simulink model "vehiclemodel_simple_empty_2020a"  (R2023b)
settings: Solver=ode23tb  StartTime=0.0  StopTime=20  FixedStep=.001  MaxStep=0.001  RelTol=1e-3  EnableMultiTasking=on
values from neighbouring files (symbols this model uses):
  a = 1.5    [truck_data_test.m]
  Ab = 0.01    [truck_data_test.m]
  ARV = 4    [truck_data_test.m]
  b = 3    [truck_data_test.m]
  Bh = 5    [truck_data_test.m]
  Bs = 10    [truck_data_test.m]
  CDV = 0.7    [truck_data_test.m]
  Ch = 2*1.2    (= 2.4)    [truck_data_test.m]
  Cs = 1.9*1.2    (= 2.28)    [truck_data_test.m]
  Dh = 0.3    [truck_data_test.m]
  Ds = 1    [truck_data_test.m]
  Eh = 1    [truck_data_test.m]
  Es = 0.97    [truck_data_test.m]
  fa = 1    [truck_data_test.m]
  ff = 1    [truck_data_test.m]
  g = 9.81    [truck_data_test.m]
  hs = 0.20    (= 0.2)    [truck_data_test.m]
  Ms = 7000    [truck_data_test.m]
  nm = 1    [truck_data_test.m]
  ntire = 10    [truck_data_test.m]
  P_s = 8e5    (= 800000)    [truck_data_test.m]
  Patm = 101356    [truck_data_test.m]
  Po = 50e3    (= 50000)    [truck_data_test.m]
  pr = 1.225    [truck_data_test.m]
  rs1 = rw1    (= 0.4)    [truck_data_test.m]
  Rw = rw1    (= 0.4)    [truck_data_test.m]
  T = 2.5    [truck_data_test.m]
  Vox = intVEL    (= 20)    [truck_data_test.m]
  WBF = 4    [truck_data_test.m]
  wp = 1/(2*(tan(wang/2)))    [truck_data_test.m]
  wr = 0.4    [truck_data_test.m]
  Xtire = 20    [truck_data_test.m]
settings Model: Creator=Abdul Moiz Awan  LastModifiedBy=yusufcagriogut
settings SolverCC: ZeroCrossControl=EnableAll  ZeroCrossAlgorithm=Adaptive  AlgebraicLoopSolver=TrustRegion
settings DataIOCC: LimitDataPoints=on  MaxDataPoints=10000
settings OptimizationCC: LifeSpan=inf
settings DebuggingCC: UnconnectedInputMsg=warning  UnconnectedOutputMsg=warning  UnconnectedLineMsg=warning  AllowSymbolicDim=off  SFUnexpectedBacktrackingDiag=warning  SFNoUnconditionalDefaultTransitionDiag=warning  SFExecutionAtInitializationDiag=none  ArithmeticOperatorsInVariantConditions=warning
settings ModelReferenceCC: EnableRefExpFcnMdlSchedulingChecks=on
settings SFSimCC: SimUseLocalCustomCode=off  CustomCodeUndefinedFunction=UseInterfaceOnly
settings RTWCC: RTWUseLocalCustomCode=off
settings CodeAppCC: StateflowObjectComments=on
settings GRTTargetCC: TargetLangStandard=C89/C90 (ANSI)
settings ConfigComp: CovMetricSettings=dw  CovSaveCumulativeToWorkspaceVar=on  CovSaveSingleToWorkspaceVar=on  CovExternalEMLEnable=off  CovSFcnEnable=off
settings SimscapeCC: SimscapeLogType=all  SimscapeLogSimulationStatistics=on  SimscapeLogDataHistory=10000

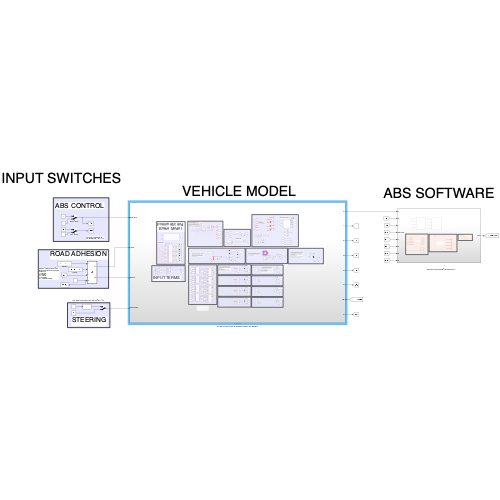
[thumbnail: Simulink's stored preview of the top-level diagram]
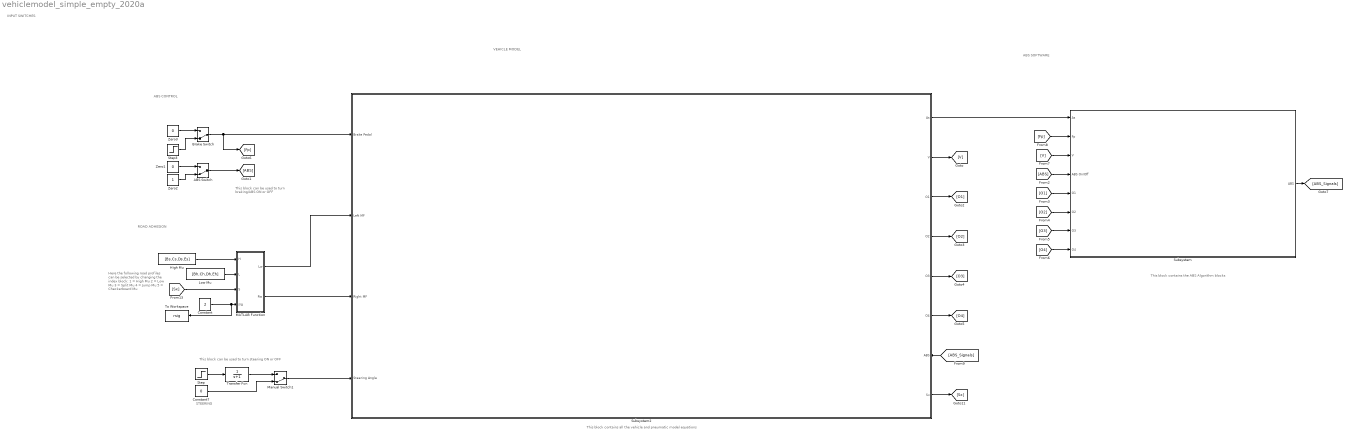
== system vehiclemodel_simple_empty_2020a ==
  note: Here the following road profiles
      | can be selected by changing the
      | index block:
      | 1 = High Mu
      | 2 = Low Mu
      | 3 = Split Mu
      | 4 = Jump Mu
      | 5 = Checkerboard Mu
  note: ABS CONTROL
  note: VEHICLE MODEL
  note: ROAD ADHESION
  note: ABS SOFTWARE
  note: INPUT SWITCHES
  note: STEERING
  note: This block contains the ABS Algorithm blocks
  note: This block contains all the vehicle and pneumatic model equations
  note: This block can be used to turn steering ON or OFF
  note: This block can be used to
      | turn braking/ABS ON or OFF
  ABS Switch : ManualSwitch  CurrentSetting=0
  Brake Switch : ManualSwitch  CurrentSetting=0
  Constant : Constant  Value=2
  Constant7 : Constant  Value=0
  High Mu : Constant  Value=[Bs,Cs,Ds,Es]
  Low Mu : Constant  Value=[Bh,Ch,Dh,Eh]
  MATLAB Function : MATLAB Function  TreatAsAtomicUnit=on
  Manual Switch1 : ManualSwitch  CurrentSetting=0
  Step : Step  After=deg2rad(3)  SampleTime=0
  Step3 : Step  SampleTime=0
  Subsystem : Subsystem
  Subsystem2 : Subsystem
      settings: PortSchema="{\"entries\":[{\"content\":{\"sides\":[{\"content\":{\"connectorIds\":[\"In1\",\"In2\",\"In3\",\"In4\"]},\"type\":\"ConnectorPlacement.EquallySpacedRectSide\",\"uuid\":\"8e59d40e-014f-4f71-bd3c-8a56eaa9320b\"},{\"content\":{\"connectorIds\":[\"Out1\",\"Out2\",\"Out3\",\"Out4\",\"Out5\",\"Out6\",\"In5\",\"Out7\"],\"side\":\"RIGHT\"},\"type\":\"ConnectorPlacement.EquallySpacedRectSide\",\"uuid\":\"f787145f-ddea-4867-9ee8-cb71aff46f3c\"},{\"content\":{\"side\":\"TOP\"},\"type\":\"ConnectorPlacement.EquallySpacedRectSide\",\"uuid\":\"5155c75c-b431-498b-ab23-6aa92088c174\"},{\"content\":{\"side\":\"BOTTOM\"},\"type\":\"ConnectorPlacement.EquallySpacedRectSide\",\"uuid\":\"2f8d0388-20b7-4bc4-84a6-56d75173057c\"}]},\"type\":\"ConnectorPlacement.EquallySpacedConnector\",\"uuid\":\"a4266be2-998a-4783-9e32-f9f9cb8c25f7\"}],\"packageUris\":[\"http://schema.mathworks.com/mf0/Connector/R2020b\"],\"version\":\"1.0\"}"
  To Workspace : ToWorkspace  VariableName=rsig  SaveFormat=Timeseries  SampleTime=-1
  Transfer Fcn : TransferFcn  Denominator=[1 1]
  Zero1 : Constant  Value=0  OutDataTypeStr=Inherit: Inherit via back propagation
  Zero2 : Constant  OutDataTypeStr=Inherit: Inherit via back propagation
  Zero3 : Constant  Value=0  OutDataTypeStr=Inherit: Inherit via back propagation
  wires:
  Zero3/1 -> Brake Switch/1
  Brake Switch/1 -> [Fp], Subsystem2/1(Brake Pedal)
  Zero1/1 -> ABS Switch/1
  Zero2/1 -> ABS Switch/2
  Step3/1 -> Brake Switch/2
  Subsystem2/2(V) -> [V]
  ABS Switch/1 -> [ABS]
  [ABS] -> Subsystem/4(ABS On/Off)
  Subsystem2/3(O1) -> [O1]
  Subsystem2/4(O2) -> [O2]
  Subsystem2/5(O3) -> [O3]
  Subsystem2/6(O4) -> [O4]
  [O1] -> Subsystem/5(O1)
  [O2] -> Subsystem/6(O2)
  [O3] -> Subsystem/7(O3)
  [O4] -> Subsystem/8(O4)
  [V] -> Subsystem/3(V)
  [Fp] -> Subsystem/2(Fp)
  Subsystem/1(ABS) -> [ABS_Signals]
  [ABS_Signals] -> Subsystem2/5(ABS)
  Step/1 -> Transfer Fcn/1
  Constant7/1 -> Manual Switch1/2
  Transfer Fcn/1 -> Manual Switch1/1
  Manual Switch1/1 -> Subsystem2/4(Steering Angle)
  MATLAB Function/2(Rw) -> Subsystem2/3(Right MF)
  Subsystem2/7(Sx) -> [Sx]
  Subsystem2/1(As) -> Subsystem/1(As)
  High Mu/1 -> MATLAB Function/1(H)
  Low Mu/1 -> MATLAB Function/2(L)
  [Sx] -> MATLAB Function/3(S)
  Constant/1 -> To Workspace/1, MATLAB Function/4(sig)
  MATLAB Function/1(Lw) -> Subsystem2/2(Left MF)

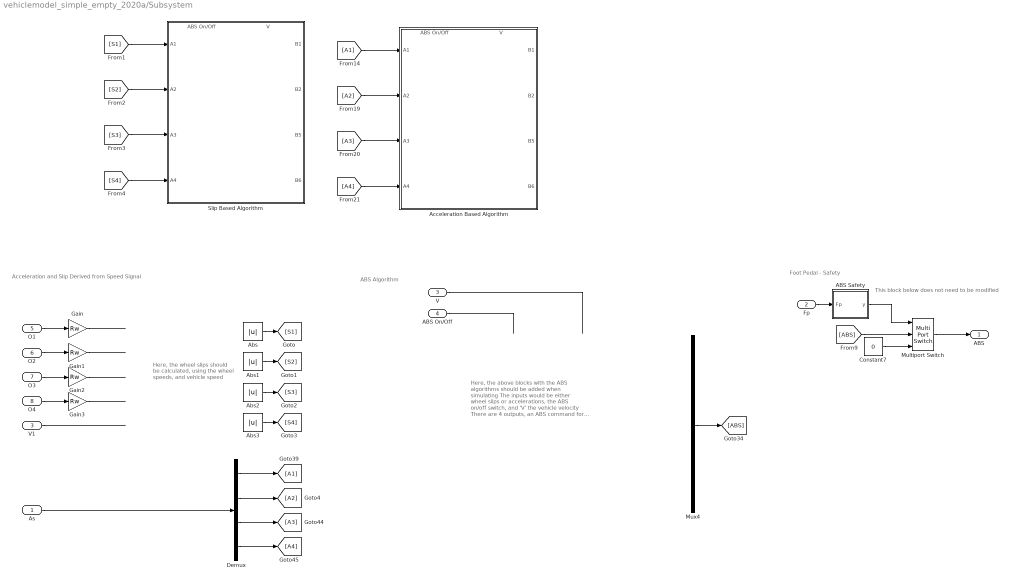
== system vehiclemodel_simple_empty_2020a/Subsystem ==
  note: Here, the wheel slips
      | should be calculated,
      | using the wheel speeds,
      | and vehicle speed
  note: Foot Pedal - Safety
  note: Acceleration and Slip Derived from Speed Signal
  note: ABS Algorithm
  note: Here, the above blocks
      | with the ABS algorithms
      | should be added when simulating
      |
      | The inputs would be either wheel
      | slips or accelerations, the ABS on/off
      | switch, and 'V' the vehicle velocity
      |
      | There are 4 outputs, an ABS command
      | for each wheel
  note: This block below does not need to be modified
  As : Inport
  Fp : Inport  Port=2
  V : Inport  Port=3
  ABS On/Off : Inport  Port=4
  O1 : Inport  Port=5
  O2 : Inport  Port=6
  O3 : Inport  Port=7
  O4 : Inport  Port=8
  ABS Safety : MATLAB Function  TreatAsAtomicUnit=on
  Abs{,1..3} (4 alike) : Abs  SaturateOnIntegerOverflow=off
  Acceleration Based Algorithm : Subsystem
      settings: PortSchema="{\"entries\":[{\"content\":{\"sides\":[{\"content\":{\"connectorIds\":[\"In1\",\"In2\",\"In3\",\"In4\"]},\"type\":\"ConnectorPlacement.EquallySpacedRectSide\",\"uuid\":\"0cf54bfd-7e95-4e49-acd0-cde280c9a58c\"},{\"content\":{\"connectorIds\":[\"Out1\",\"Out2\",\"Out3\",\"Out4\"],\"side\":\"RIGHT\"},\"type\":\"ConnectorPlacement.EquallySpacedRectSide\",\"uuid\":\"586cf5cf-8639-456b-b48e-ff3e77509e66\"},{\"content\":{\"connectorIds\":[\"In5\",\"In6\"],\"side\":\"TOP\"},\"type\":\"ConnectorPlacement.EquallySpacedRectSide\",\"uuid\":\"7bf15eda-a81d-4bd7-ab4e-9ac22b0c7db2\"}]},\"type\":\"ConnectorPlacement.EquallySpacedConnector\",\"uuid\":\"c618e342-5041-438f-9a1b-df95de83ed7e\"}],\"packageUris\":[\"http://schema.mathworks.com/mf0/Connector/R2020b\"],\"version\":\"1.0\"}"
  Constant7 : Constant  Value=0
  Demux : Demux
  Gain{,1..3} (4 alike) : Gain  Gain=Rw
  Multiport Switch : MultiPortSwitch  Inputs=2  SaturateOnIntegerOverflow=off  InputSameDT=off
  Mux4 : Mux
  Slip Based Algorithm : Subsystem
      settings: PortSchema="{\"entries\":[{\"content\":{\"sides\":[{\"content\":{\"connectorIds\":[\"In1\",\"In2\",\"In3\",\"In4\"]},\"type\":\"ConnectorPlacement.EquallySpacedRectSide\",\"uuid\":\"0cf54bfd-7e95-4e49-acd0-cde280c9a58c\"},{\"content\":{\"connectorIds\":[\"Out1\",\"Out2\",\"Out3\",\"Out4\"],\"side\":\"RIGHT\"},\"type\":\"ConnectorPlacement.EquallySpacedRectSide\",\"uuid\":\"586cf5cf-8639-456b-b48e-ff3e77509e66\"},{\"content\":{\"connectorIds\":[\"In5\",\"In6\"],\"side\":\"TOP\"},\"type\":\"ConnectorPlacement.EquallySpacedRectSide\",\"uuid\":\"7bf15eda-a81d-4bd7-ab4e-9ac22b0c7db2\"}]},\"type\":\"ConnectorPlacement.EquallySpacedConnector\",\"uuid\":\"c618e342-5041-438f-9a1b-df95de83ed7e\"}],\"packageUris\":[\"http://schema.mathworks.com/mf0/Connector/R2020b\"],\"version\":\"1.0\"}"
  V1 : InportShadow  Port=3
  ABS : Outport
  wires:
  V/1 -> ?
  ? -> Mux4/4
  ? -> Mux4/2
  ABS On/Off/1 -> ?
  [ABS] -> Multiport Switch/2
  ? -> Mux4/1
  Mux4/1 -> [ABS]
  ? -> Mux4/3
  Constant7/1 -> Multiport Switch/3
  ABS Safety/1(y) -> Multiport Switch/1
  Fp/1 -> ABS Safety/1(Fp)
  Multiport Switch/1 -> ABS/1
  V1/1 -> ?
  Gain/1 -> ?
  Gain1/1 -> ?
  Gain2/1 -> ?
  Gain3/1 -> ?
  Abs/1 -> [S1]
  Abs1/1 -> [S2]
  Abs2/1 -> [S3]
  Demux/4 -> [A4]
  O4/1 -> Gain3/1
  Demux/1 -> [A1]
  O1/1 -> Gain/1
  O2/1 -> Gain1/1
  O3/1 -> Gain2/1
  Demux/2 -> [A2]
  Demux/3 -> [A3]
  As/1 -> Demux/1
  [A4] -> Acceleration Based Algorithm/4(A4)
  [A3] -> Acceleration Based Algorithm/3(A3)
  [A2] -> Acceleration Based Algorithm/2(A2)
  [A1] -> Acceleration Based Algorithm/1(A1)
  Abs3/1 -> [S4]
  [S1] -> Slip Based Algorithm/1(A1)
  [S2] -> Slip Based Algorithm/2(A2)
  [S3] -> Slip Based Algorithm/3(A3)
  [S4] -> Slip Based Algorithm/4(A4)

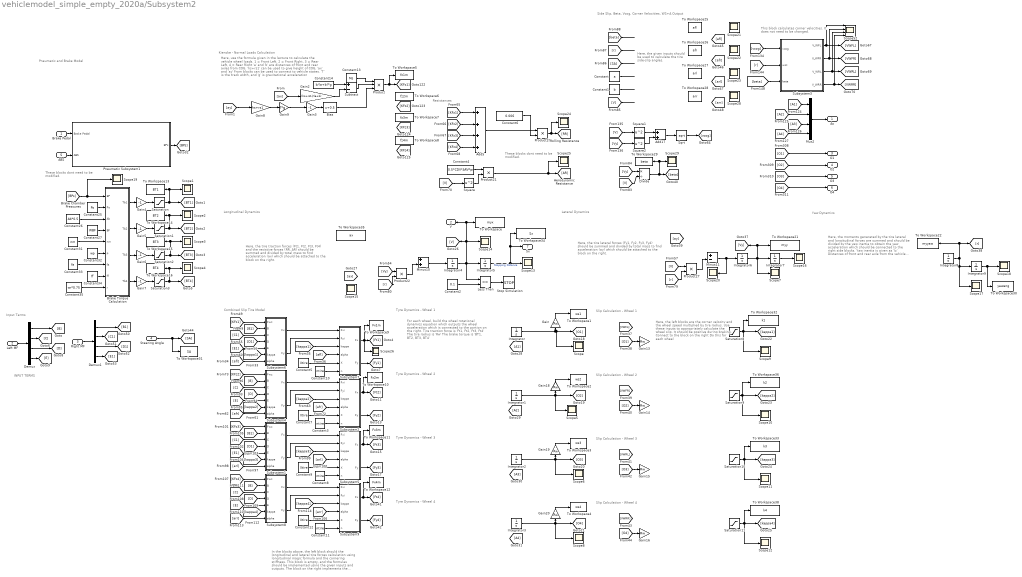
== system vehiclemodel_simple_empty_2020a/Subsystem2 ==
  note: This block calculates corner velocities.
      | It does not need to be changed.
  note: These blocks dont
      | need to be modified.
  note: Combined Slip Tire Model
  note: Side Slip, Beta, Vcog, Corner Velocities, WS+A Output
  note: Yaw Dynamics
  note: Lateral Dynamics
  note: Resistances
  note: Input Terms
  note: Pneumatic and Brake Model
  note: INPUT TERMS
  note: Kiencke - Normal Loads Calculation
  note: Tyre Dynamics - Wheel 1
  note: Tyre Dynamics - Wheel 2
  note: Tyre Dynamics - Wheel 3
  note: Tyre Dynamics - Wheel 4
  note: Slip Calculation - Wheel 1
  note: Slip Calculation - Wheel 2
  note: Slip Calculation - Wheel 3
  note: Slip Calculation - Wheel 4
  note: Longitudinal Dynamics
  note: In the blocks above, the left block should
      | the longitudinal and lateral tire forces calculation
      | using longitudinal magic formula and the
      | cornering stiffness. This block is empty, and the
      | formulas should be implemented using the given
      | inputs and outputs.
      |
      | The block on the right implements the combined
      | slip model and does not need to be modified.
  note: For each wheel, build the wheel rotational
      | dynamics equation which outputs the wheel
      | acceleration which is connected to the portion
      | on the right.
      |
      | Tire traction force is 'Ft1, Ft2, Ft3, Ft4'
      | The tire radius is 'Rw'
      | The brake torque is 'BT1, BT2, BT3, BT4'
  note: Here, the left blocks are the corner velocity
      | and the wheel speed multiplied by tire
      | radius. Use these inputs to appropriately
      | calculate the wheel slip.
      |
      | It should be positive during braking. Connect
      | to the block on the right
      |
      | Do this for each wheel
  note: Here, the tire traction forces (Ft1, Ft2, Ft3, Ft4)
      | and the resistive forces (RR, AR) should be
      | summed and divided by total mass to find
      | acceleration (ax) which should be attached to
      | the block on the right.
  note: Here, the tire lateral forces (Fy1, Fy2, Fy3, Fy4)
      | should be summed and divided by total mass
      | to find acceleration (ay) which should be attached
      | to the block on the right.
  note: Here, the moments generated by the tire lateral
      | and longitudinal forces are summed and should
      | be divided by the yaw inertia to obtain the yaw
      | acceleration which should be connected to the
      | right side blocks.
      |
      | Yaw inertia is given as 'Iz'
      |
      | Distances of front and rear axle from the vehicle
      | COG are given as 'a' and 'b' respectively.
  note: Here, use the formula given in the lecture to
      | calculate the vehicle wheel loads.
      | 1 = Front Left, 2 = Front Right, 3 = Rear Left, 4 = Rear Right
      |
      | 'a' and 'b' are distances of front and rear axles from COG,
      | 'hs+rs1' can be used to give height of COG,
      | 'ax' and 'ay' From blocks can be used to connect to vehicle
      | states.
      | 'T' is the track width, and 'g' is gravitational acceleration
  note: These blocks dont
      | need to be modified.
  note: Here, the given
      | inputs should
      | be used to calculate
      | the tire side-slip angles.
  Brake Pedal : Inport
  Left MF : Inport  Port=2
  Right MF : Inport  Port=3
  Steering Angle : Inport  Port=4
  ABS : Inport  Port=5
  Add17 : Sum
  Add5 : Sum  Inputs=++++
  Bias : Bias  Bias=0.5  SaturateOnIntegerOverflow=off
  Brake Torque Calculation : MATLAB Function  TreatAsAtomicUnit=on
  Constant : Constant  Value=a
  Constant1 : Constant  Value=b
  Constant{3,8,10..11} (4 alike) : Constant  Value=ntire
  Constant{5,7,9,12} (4 alike) : Constant  Value=Xtire
  Constant13 : Constant  Value=Ms
  Constant14 : Constant  Value=b/(a+b)*g
  Constant2 : Constant  Value=0.1
  Constant25 : Constant  Value=Po
  Constant26 : Constant  Value=Ab*0.5
  Constant27 : Constant  Value=WBF
  Constant31 : Constant  Value=nm
  Constant32 : Constant  Value=wp
  Constant33 : Constant  Value=fa
  Constant34 : Constant  Value=ff
  Constant35 : Constant  Value=wr*0.75
  Constant4 : Constant  Value=0.5*CDV*ARV*pr
  Constant6 : Constant  Value=0.006
  Demux : Demux
  Demux1 : Demux
  Divide : Product  Inputs=*/
  Gain{,13..16,18..20} (8 alike) : Gain  Gain=Rw
  Gain2 : Gain  Gain=(hs+rs1)/(a+b)
  Gain{3..7} (5 alike) : Gain  Gain=-1
  Gain8 : Gain  Gain=hs+rs1
  Gain9 : Gain  Gain=T*g
  Integrator{,1..3} (4 alike) : Integrator  InitialCondition=Vox/Rw  LimitOutput=on  LowerSaturationLimit=0
  Integrator4 : Integrator  InitialCondition=Vox
  Integrator{5..9} (5 alike) : Integrator
  Less Than : RelationalOperator  Operator=<=  OutDataTypeStr=boolean  RndMeth=Simplest  InputSameDT=off
  Minus10 : Sum
  Minus11 : Sum  Inputs=+-
  Mux2 : Mux
  Pneumatic Subsystem1 : Subsystem
  Product : Product  Inputs=3
  Product{20..22,27} (4 alike) : Product
  Saturation{,1..3} (4 alike) : Saturate  UpperLimit=0  LowerLimit=-inf
  Saturation{8..11} (4 alike) : Saturate  UpperLimit=1  LowerLimit=-1
  Scope{,1..26,28..29} (29 alike) : Scope
  Scope52 : Scope  NumInputPorts=4
  Sqrt : Sqrt
  Square : Math  Operator=square
  Square1 : Math  Operator=square
  Square2 : Math  Operator=square
  Stop Simulation : Stop
  Subsystem1 : Subsystem
  Subsystem2 : Subsystem
  Subsystem3 : Subsystem
  Subsystem4 : Subsystem
  Subsystem5 : Subsystem
  Subsystem6 : Subsystem
  Subsystem7 : Subsystem
  Subsystem8 : Subsystem
  Subsystem9 : Subsystem
  Subtract : Sum  Inputs=+-
  To Workspace : ToWorkspace  VariableName=myx  SaveFormat=Timeseries  SampleTime=-1
  To Workspace1 : ToWorkspace  VariableName=ws1  SaveFormat=Timeseries  SampleTime=-1
  To Workspace10 : ToWorkspace  VariableName=Fx2m  SaveFormat=Timeseries  SampleTime=-1
  To Workspace11 : ToWorkspace  VariableName=Fx3m  SaveFormat=Timeseries  SampleTime=-1
  To Workspace12 : ToWorkspace  VariableName=Fx4m  SaveFormat=Timeseries  SampleTime=-1
  To Workspace13 : ToWorkspace  VariableName=BT1  SaveFormat=Timeseries  SampleTime=-1
  To Workspace14 : ToWorkspace  VariableName=BT2  SaveFormat=Timeseries  SampleTime=-1
  To Workspace15 : ToWorkspace  VariableName=BT3  SaveFormat=Timeseries  SampleTime=-1
  To Workspace16 : ToWorkspace  VariableName=BT4  SaveFormat=Timeseries  SampleTime=-1
  To Workspace2 : ToWorkspace  VariableName=ws2  SaveFormat=Timeseries  SampleTime=-1
  To Workspace21 : ToWorkspace  VariableName=myy  SaveFormat=Timeseries  SampleTime=-1
  To Workspace22 : ToWorkspace  VariableName=myyaw  SaveFormat=Timeseries  SampleTime=-1
  To Workspace25 : ToWorkspace  VariableName=afl  SaveFormat=Timeseries  SampleTime=-1
  To Workspace26 : ToWorkspace  VariableName=afr  SaveFormat=Timeseries  SampleTime=-1
  To Workspace27 : ToWorkspace  VariableName=arl  SaveFormat=Timeseries  SampleTime=-1
  To Workspace28 : ToWorkspace  VariableName=arr  SaveFormat=Timeseries  SampleTime=-1
  To Workspace29 : ToWorkspace  VariableName=beta  SaveFormat=Timeseries  SampleTime=-1
  To Workspace3 : ToWorkspace  VariableName=ws3  SaveFormat=Timeseries  SampleTime=-1
  To Workspace30 : ToWorkspace  VariableName=yawang  SaveFormat=Timeseries  SampleTime=-1
  To Workspace31 : ToWorkspace  VariableName=SA  SaveFormat=Timeseries  SampleTime=-1
  To Workspace32 : ToWorkspace  VariableName=k1  SaveFormat=Timeseries  SampleTime=-1
  To Workspace33 : ToWorkspace  VariableName=k3  SaveFormat=Timeseries  SampleTime=-1
  To Workspace34 : ToWorkspace  VariableName=Sx  SaveFormat=Timeseries  SampleTime=-1
  To Workspace35 : ToWorkspace  VariableName=ax  SaveFormat=Timeseries  SampleTime=-1
  To Workspace36 : ToWorkspace  VariableName=k2  SaveFormat=Timeseries  SampleTime=-1
  To Workspace38 : ToWorkspace  VariableName=k4  SaveFormat=Timeseries  SampleTime=-1
  To Workspace4 : ToWorkspace  VariableName=ws4  SaveFormat=Timeseries  SampleTime=-1
  To Workspace5 : ToWorkspace  VariableName=fz1m  SaveFormat=Timeseries  SampleTime=-1
  To Workspace6 : ToWorkspace  VariableName=fz2m  SaveFormat=Timeseries  SampleTime=-1
  To Workspace7 : ToWorkspace  VariableName=fz3m  SaveFormat=Timeseries  SampleTime=-1
  To Workspace8 : ToWorkspace  VariableName=fz4m  SaveFormat=Timeseries  SampleTime=-1
  To Workspace9 : ToWorkspace  VariableName=Fx1m  SaveFormat=Timeseries  SampleTime=-1
  As : Outport
  V : Outport  Port=2
  O1 : Outport  Port=3
  O2 : Outport  Port=4
  O3 : Outport  Port=5
  O4 : Outport  Port=6
  Sx : Outport  Port=7
  wires:
  Brake Pedal/1 -> Pneumatic Subsystem1/1(Brake Pedal)
  ? -> To Workspace8/1, [KFz4]
  ? -> To Workspace7/1, [KFz3]
  ? -> To Workspace6/1, [KFz2]
  Brake Torque Calculation/4(Tb4) -> Gain7/1
  Gain5/1 -> Saturation1/1
  Gain4/1 -> Saturation/1
  Constant27/1 -> Brake Torque Calculation/4(BF)
  Constant26/1 -> Brake Torque Calculation/3(Ab)
  Gain6/1 -> Saturation2/1
  Brake Torque Calculation/3(Tb3) -> Gain6/1
  Constant31/1 -> Brake Torque Calculation/5(nm)
  Constant33/1 -> Brake Torque Calculation/7(fa)
  Gain7/1 -> Saturation3/1
  Constant35/1 -> Brake Torque Calculation/9(r)
  Brake Torque Calculation/1(Tb1) -> Gain4/1
  Constant32/1 -> Brake Torque Calculation/6(p)
  Brake Torque Calculation/2(Tb2) -> Gain5/1
  Constant25/1 -> Brake Torque Calculation/2(Po)
  Constant34/1 -> Brake Torque Calculation/8(ff)
  Saturation/1 -> [BT1], Scope1/1, To Workspace13/1
  Saturation1/1 -> [BT2], Scope2/1, To Workspace14/1
  Saturation3/1 -> [BT4], Scope4/1, To Workspace16/1
  Pneumatic Subsystem1/1(BPs) -> [BPs]
  Left MF/1 -> Demux/1
  Demux/1 -> [B]
  Demux/2 -> [C]
  Demux/3 -> [D]
  Demux/4 -> [E]
  Integrator/1 -> [O1], Scope/1, Gain/1
  ? -> [A1], Integrator/1
  ? -> Integrator1/1, [A2]
  Integrator1/1 -> [O2], Scope5/1, Gain18/1
  Integrator2/1 -> [O3], Scope6/1, Gain19/1
  ? -> Integrator2/1, [A3]
  ? -> Integrator3/1, [A4]
  Integrator3/1 -> [O4], Scope8/1, Gain20/1
  Saturation8/1 -> Scope9/1, To Workspace32/1, [kappa1]
  [O1] -> Gain13/1
  [O2] -> Gain14/1
  Saturation9/1 -> To Workspace36/1, Scope10/1, [kappa2]
  Saturation10/1 -> Scope11/1, To Workspace33/1, [kappa3]
  [O3] -> Gain15/1
  [O4] -> Gain16/1
  Saturation11/1 -> To Workspace38/1, Scope12/1, [kappa4]
  Integrator5/1 -> To Workspace34/1, Sx/1, Scope13/1  "Stopping Dstance"
  Less Than/1 -> Stop Simulation/1
  Constant2/1 -> Less Than/2
  Integrator4/1 -> Less Than/1, To Workspace/1, V/1, Scope14/1, [V], Integrator5/1
  ? -> To Workspace35/1, Scope15/1, [ax], Minus10/1
  Gain/1 -> To Workspace1/1
  Gain18/1 -> To Workspace2/1
  Gain19/1 -> To Workspace3/1
  Gain20/1 -> To Workspace4/1
  Add5/1 -> Product20/1
  [KFz4] -> Add5/4
  [KFz3] -> Add5/3
  [KFz2] -> Add5/2
  [KFz1] -> Add5/1
  Product20/1 -> Scope24/1, [RR]
  Constant4/1 -> Product21/1
  [V] -> Square/1
  Square/1 -> Product21/2
  Product21/1 -> Scope25/1, [AR]
  Constant6/1 -> Product20/2
  Product/1 -> To Workspace5/1, [KFz1]
  [O3] -> O3/1
  [O2] -> O2/1
  [O4] -> O4/1
  [O1] -> O1/1
  ABS/1 -> Pneumatic Subsystem1/2(ABS)
  Product22/1 -> Minus10/2
  Product27/1 -> Minus11/2
  ? -> Minus11/1, [ay]
  Minus11/1 -> Scope20/1, Integrator6/1
  Integrator6/1 -> To Workspace21/1, [Vy], Scope7/1, Integrator7/1
  Integrator7/1 -> Scope16/1
  [Vy] -> Product22/1
  [V] -> Product27/1
  ? -> Integrator8/1
  Integrator8/1 -> Scope17/1, Integrator9/1, To Workspace22/1, [r]
  Integrator9/1 -> Scope18/1, To Workspace30/1
  [r] -> Product27/2
  [r] -> Product22/2
  [Vy] -> Divide/1
  [V] -> Divide/2
  Divide/1 -> Scope29/1, To Workspace29/1, [beta]
  Steering Angle/1 -> To Workspace31/1, [SA]
  Constant/1 -> ?
  Constant1/1 -> ?
  [V] -> ?
  [SA] -> ?
  [r] -> ?
  [beta] -> ?
  ? -> To Workspace25/1, Scope21/1, [afl]  "From Formula"
  ? -> To Workspace26/1, Scope22/1, [afr]  "From Fomula"
  ? -> To Workspace27/1, Scope23/1, [arl]  "From Formula"
  ? -> Scope28/1, To Workspace28/1, [arr]  "From Formula"
  Right MF/1 -> Demux1/1
  Minus10/1 -> Integrator4/1
  [BPs] -> Scope19/1, Brake Torque Calculation/1(BP)
  [A2] -> Mux2/2
  [A1] -> Mux2/1
  [A3] -> Mux2/3
  [A4] -> Mux2/4
  Mux2/1 -> As/1
  Subsystem3/4(V_WRR) -> Scope52/4, [VWRR]
  Subsystem3/2(V_WFR) -> Scope52/2, [VWFR]
  [vcog] -> Subsystem3/1(vcog)
  [r] -> Subsystem3/2(wsz)
  [beta] -> Subsystem3/3(beta)
  Subsystem3/3(V_WRL) -> Scope52/3, [VWRL]
  Subsystem3/1(V_WFL) -> Scope52/1, [VWFL]
  [V] -> Square1/1
  [Vy] -> Square2/1
  Square1/1 -> Add17/1
  Square2/1 -> Add17/2
  Add17/1 -> Sqrt/1
  Sqrt/1 -> [vcog]
  Demux1/1 -> [B1]
  Demux1/2 -> [C1]
  Demux1/3 -> [D1]
  Demux1/4 -> [E1]
  [afl] -> Subsystem7/4(alpha)
  Subsystem6/2(Fy) -> Subsystem7/2(Fyi)
  [kappa1] -> Subsystem7/3(kappa)
  Subsystem7/2(Fy) -> [Fy1]
  [C1] -> Subsystem6/3(C)
  [kappa1] -> Subsystem6/6(kappa)
  [D1] -> Subsystem6/4(D)
  [KFz1] -> Subsystem6/1(Fwz)
  [E1] -> Subsystem6/5(E)
  Constant5/1 -> Subsystem7/5(X)
  [afl] -> Subsystem6/7(alpha)
  Subsystem6/1(Fx) -> Subsystem7/1(Fxi)
  [B1] -> Subsystem6/2(B)
  Constant10/1 -> Subsystem7/6(n)
  Constant3/1 -> Subsystem2/6(n)
  [B] -> Subsystem4/2(B)
  Subsystem2/1(Fx) -> To Workspace10/1, [Ft2]
  Subsystem4/1(Fx) -> Subsystem2/1(Fxi)
  [afr] -> Subsystem4/7(alpha)
  Constant7/1 -> Subsystem2/5(X)
  [E] -> Subsystem4/5(E)
  [KFz2] -> Subsystem4/1(Fwz)
  [D] -> Subsystem4/4(D)
  [kappa2] -> Subsystem4/6(kappa)
  [C] -> Subsystem4/3(C)
  Subsystem2/2(Fy) -> [Fy2]
  [kappa2] -> Subsystem2/3(kappa)
  Subsystem4/2(Fy) -> Subsystem2/2(Fyi)
  [afr] -> Subsystem2/4(alpha)
  [arl] -> Subsystem5/4(alpha)
  Subsystem1/2(Fy) -> Subsystem5/2(Fyi)
  [kappa3] -> Subsystem5/3(kappa)
  Subsystem5/2(Fy) -> [Fy3]
  [C1] -> Subsystem1/3(C)
  [kappa3] -> Subsystem1/6(kappa)
  [D1] -> Subsystem1/4(D)
  [KFz3] -> Subsystem1/1(Fwz)
  [E1] -> Subsystem1/5(E)
  Constant9/1 -> Subsystem5/5(X)
  [arl] -> Subsystem1/7(alpha)
  Subsystem1/1(Fx) -> Subsystem5/1(Fxi)
  Subsystem5/1(Fx) -> To Workspace11/1, [Ft3]
  [B1] -> Subsystem1/2(B)
  Constant8/1 -> Subsystem5/6(n)
  Constant11/1 -> Subsystem9/6(n)
  [B] -> Subsystem8/2(B)
  Subsystem9/1(Fx) -> To Workspace12/1, [Ft4]
  Subsystem8/1(Fx) -> Subsystem9/1(Fxi)
  [arr] -> Subsystem8/7(alpha)
  Constant12/1 -> Subsystem9/5(X)
  [E] -> Subsystem8/5(E)
  [KFz4] -> Subsystem8/1(Fwz)
  [D] -> Subsystem8/4(D)
  [kappa4] -> Subsystem8/6(kappa)
  [C] -> Subsystem8/3(C)
  Subsystem9/2(Fy) -> [Fy4]
  [kappa4] -> Subsystem9/3(kappa)
  Subsystem8/2(Fy) -> Subsystem9/2(Fyi)
  [arr] -> Subsystem9/4(alpha)
  Subsystem7/1(Fx) -> To Workspace9/1, Scope26/1, [Ft1]
  Saturation2/1 -> [BT3], Scope3/1, To Workspace15/1
  Constant13/1 -> Product/1
  [ax] -> Gain2/1
  Gain2/1 -> Subtract/2
  Constant14/1 -> Subtract/1
  Subtract/1 -> Product/2
  [ay] -> Gain8/1
  Gain8/1 -> Gain9/1
  Gain9/1 -> Gain3/1
  Bias/1 -> Product/3
  Gain3/1 -> Bias/1

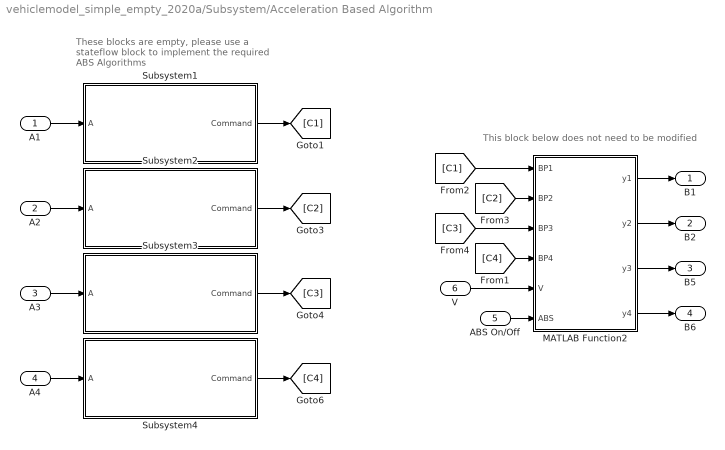
== system vehiclemodel_simple_empty_2020a/Subsystem/Acceleration Based Algorithm ==
  note: This block below does not need to be modified
  note: These blocks are empty, please use
      | a stateflow block to implement the required
      | ABS Algorithms
  A1 : Inport
  A2 : Inport  Port=2
  A3 : Inport  Port=3
  A4 : Inport  Port=4
  ABS On/Off : Inport  Port=5
  V : Inport  Port=6
  MATLAB Function2 : MATLAB Function  TreatAsAtomicUnit=on
  Subsystem1 : Subsystem
  Subsystem2 : Subsystem
  Subsystem3 : Subsystem
  Subsystem4 : Subsystem
  B1 : Outport
  B2 : Outport  Port=2
  B5 : Outport  Port=3
  B6 : Outport  Port=4
  wires:
  A4/1 -> Subsystem4/1(A)
  A3/1 -> Subsystem3/1(A)
  Subsystem3/1(Command) -> [C3]
  Subsystem4/1(Command) -> [C4]
  A2/1 -> Subsystem2/1(A)
  A1/1 -> Subsystem1/1(A)
  Subsystem1/1(Command) -> [C1]
  Subsystem2/1(Command) -> [C2]
  ABS On/Off/1 -> MATLAB Function2/6(ABS)
  MATLAB Function2/1(y1) -> B1/1
  V/1 -> MATLAB Function2/5(V)
  MATLAB Function2/2(y2) -> B2/1
  MATLAB Function2/4(y4) -> B6/1
  MATLAB Function2/3(y3) -> B5/1
  [C1] -> MATLAB Function2/1(BP1)
  [C2] -> MATLAB Function2/2(BP2)
  [C3] -> MATLAB Function2/3(BP3)
  [C4] -> MATLAB Function2/4(BP4)

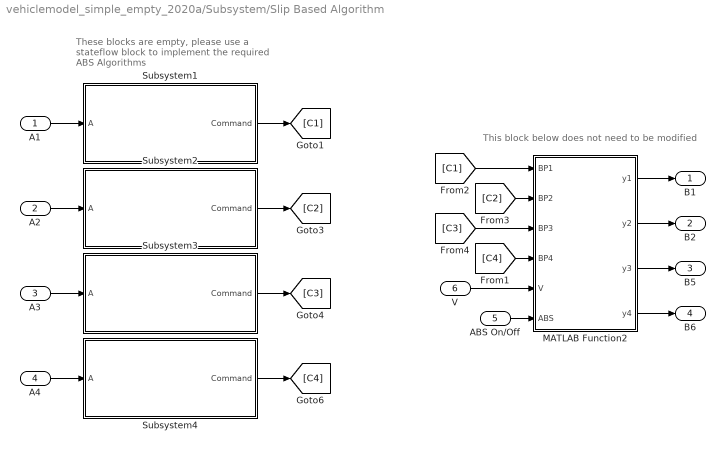
== system vehiclemodel_simple_empty_2020a/Subsystem/Slip Based Algorithm ==
  note: These blocks are empty, please use
      | a stateflow block to implement the required
      | ABS Algorithms
  note: This block below does not need to be modified
  A1 : Inport
  A2 : Inport  Port=2
  A3 : Inport  Port=3
  A4 : Inport  Port=4
  ABS On/Off : Inport  Port=5
  V : Inport  Port=6
  MATLAB Function2 : MATLAB Function  TreatAsAtomicUnit=on
  Subsystem1 : Subsystem
  Subsystem2 : Subsystem
  Subsystem3 : Subsystem
  Subsystem4 : Subsystem
  B1 : Outport
  B2 : Outport  Port=2
  B5 : Outport  Port=3
  B6 : Outport  Port=4
  wires:
  [C4] -> MATLAB Function2/4(BP4)
  [C3] -> MATLAB Function2/3(BP3)
  [C2] -> MATLAB Function2/2(BP2)
  [C1] -> MATLAB Function2/1(BP1)
  MATLAB Function2/3(y3) -> B5/1
  MATLAB Function2/4(y4) -> B6/1
  MATLAB Function2/2(y2) -> B2/1
  V/1 -> MATLAB Function2/5(V)
  MATLAB Function2/1(y1) -> B1/1
  ABS On/Off/1 -> MATLAB Function2/6(ABS)
  Subsystem2/1(Command) -> [C2]
  Subsystem1/1(Command) -> [C1]
  A1/1 -> Subsystem1/1(A)
  A2/1 -> Subsystem2/1(A)
  Subsystem4/1(Command) -> [C4]
  Subsystem3/1(Command) -> [C3]
  A3/1 -> Subsystem3/1(A)
  A4/1 -> Subsystem4/1(A)

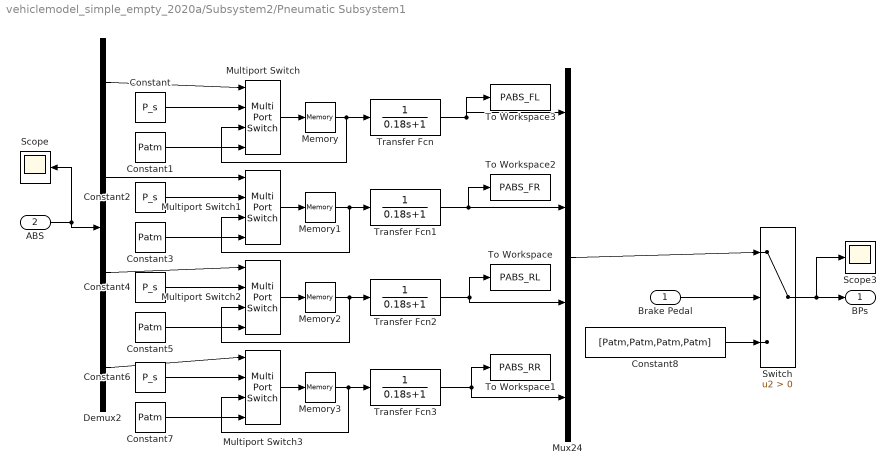
== system vehiclemodel_simple_empty_2020a/Subsystem2/Pneumatic Subsystem1 ==
  Brake Pedal : Inport
  ABS : Inport  Port=2
  Constant{,2,4,6} (4 alike) : Constant  Value=P_s
  Constant{1,3,5,7} (4 alike) : Constant  Value=Patm
  Constant8 : Constant  Value=[Patm,Patm,Patm,Patm]
  Demux2 : Demux
  Memory{,1..3} (4 alike) : Memory  InitialCondition=Patm
  Multiport Switch{,1..3} (4 alike) : MultiPortSwitch  DiagnosticForDefault=None  SaturateOnIntegerOverflow=off  InputSameDT=off
  Mux24 : Mux
  Scope : Scope
  Scope3 : Scope
  Switch : Switch  Criteria=u2 > Threshold  SaturateOnIntegerOverflow=off  InputSameDT=off
  To Workspace : ToWorkspace  VariableName=PABS_RL  SaveFormat=Timeseries  SampleTime=-1
  To Workspace1 : ToWorkspace  VariableName=PABS_RR  SaveFormat=Timeseries  SampleTime=-1
  To Workspace2 : ToWorkspace  VariableName=PABS_FR  SaveFormat=Timeseries  SampleTime=-1
  To Workspace3 : ToWorkspace  VariableName=PABS_FL  SaveFormat=Timeseries  SampleTime=-1
  Transfer Fcn{,1..3} (4 alike) : TransferFcn  Denominator=[0.18 1]
  BPs : Outport
  wires:
  Switch/1 -> Scope3/1, BPs/1
  Memory/1 -> Multiport Switch/3, Transfer Fcn/1
  Demux2/3 -> Multiport Switch2/1
  Demux2/2 -> Multiport Switch1/1
  ABS/1 -> Scope/1, Demux2/1
  Demux2/1 -> Multiport Switch/1
  Demux2/4 -> Multiport Switch3/1
  Constant/1 -> Multiport Switch/2
  Constant1/1 -> Multiport Switch/4
  Multiport Switch/1 -> Memory/1
  Multiport Switch1/1 -> Memory1/1
  Constant3/1 -> Multiport Switch1/4
  Constant2/1 -> Multiport Switch1/2
  Memory1/1 -> Multiport Switch1/3, Transfer Fcn1/1
  Memory2/1 -> Multiport Switch2/3, Transfer Fcn2/1
  Constant4/1 -> Multiport Switch2/2
  Constant5/1 -> Multiport Switch2/4
  Multiport Switch2/1 -> Memory2/1
  Multiport Switch3/1 -> Memory3/1
  Constant7/1 -> Multiport Switch3/4
  Constant6/1 -> Multiport Switch3/2
  Memory3/1 -> Multiport Switch3/3, Transfer Fcn3/1
  Transfer Fcn/1 -> To Workspace3/1, Mux24/1
  Transfer Fcn2/1 -> To Workspace/1, Mux24/3
  Transfer Fcn3/1 -> To Workspace1/1, Mux24/4
  Mux24/1 -> Switch/1
  Brake Pedal/1 -> Switch/2
  Constant8/1 -> Switch/3
  Transfer Fcn1/1 -> To Workspace2/1, Mux24/2

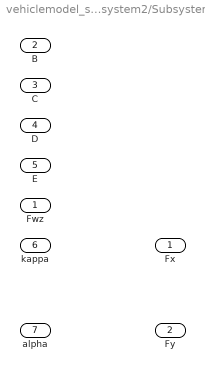
== system vehiclemodel_simple_empty_2020a/Subsystem2/Subsystem1 ==
  Fwz : Inport
  B : Inport  Port=2
  C : Inport  Port=3
  D : Inport  Port=4
  E : Inport  Port=5
  kappa : Inport  Port=6
  alpha : Inport  Port=7
  Fx : Outport
  Fy : Outport  Port=2

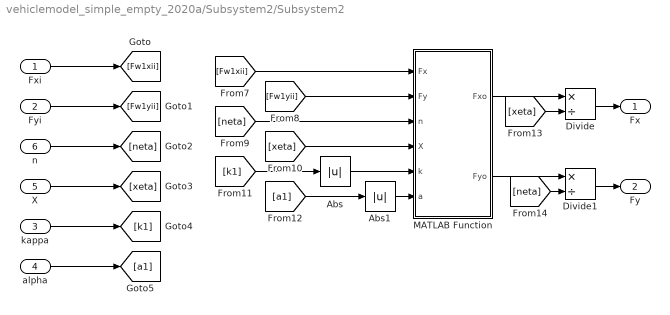
== system vehiclemodel_simple_empty_2020a/Subsystem2/Subsystem2 ==
  Fxi : Inport
  Fyi : Inport  Port=2
  kappa : Inport  Port=3
  alpha : Inport  Port=4
  X : Inport  Port=5
  n : Inport  Port=6
  Abs : Abs  SaturateOnIntegerOverflow=off
  Abs1 : Abs  SaturateOnIntegerOverflow=off
  Divide : Product  Inputs=*/
  Divide1 : Product  Inputs=*/
  MATLAB Function : MATLAB Function  TreatAsAtomicUnit=on
  Fx : Outport
  Fy : Outport  Port=2
  wires:
  Fxi/1 -> [Fw1xii]
  Fyi/1 -> [Fw1yii]
  n/1 -> [neta]
  X/1 -> [xeta]
  alpha/1 -> [a1]
  kappa/1 -> [k1]
  Divide/1 -> Fx/1
  [Fw1xii] -> MATLAB Function/1(Fx)
  [k1] -> Abs/1
  [neta] -> MATLAB Function/3(n)
  [Fw1yii] -> MATLAB Function/2(Fy)
  MATLAB Function/1(Fxo) -> Divide/1
  Abs1/1 -> MATLAB Function/6(a)
  [xeta] -> MATLAB Function/4(X)
  [a1] -> Abs1/1
  [xeta] -> Divide/2
  Abs/1 -> MATLAB Function/5(k)
  MATLAB Function/2(Fyo) -> Divide1/1
  [neta] -> Divide1/2
  Divide1/1 -> Fy/1

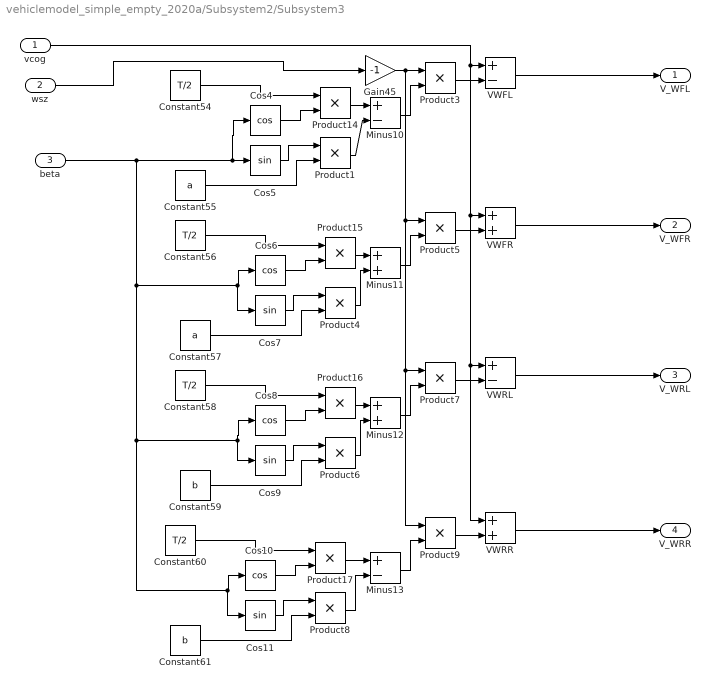
== system vehiclemodel_simple_empty_2020a/Subsystem2/Subsystem3 ==
  vcog : Inport
  wsz : Inport  Port=2
  beta : Inport  Port=3
  Constant{54,56,58,60} (4 alike) : Constant  Value=T/2
  Constant55 : Constant  Value=a
  Constant57 : Constant  Value=a
  Constant59 : Constant  Value=b
  Constant61 : Constant  Value=b
  Cos{4,6,8,10} (4 alike) : Trigonometry  Operator=cos
  Cos{5,7,9,11} (4 alike) : Trigonometry
  Gain45 : Gain  Gain=-1
  Minus10 : Sum  Inputs=+-
  Minus11 : Sum
  Minus12 : Sum
  Minus13 : Sum  Inputs=+-
  Product{1,3..9,14..17} (12 alike) : Product
  VWFL : Sum  Inputs=+-
  VWFR : Sum
  VWRL : Sum  Inputs=+-
  VWRR : Sum
  V_WFL : Outport
  V_WFR : Outport  Port=2
  V_WRL : Outport  Port=3
  V_WRR : Outport  Port=4
  wires:
  VWFR/1 -> V_WFR/1
  Constant57/1 -> Product4/2
  Minus12/1 -> Product7/2
  Cos9/1 -> Product6/1
  Product1/1 -> Minus10/2
  Product6/1 -> Minus12/2
  Product16/1 -> Minus12/1
  Constant56/1 -> Product15/1
  Product4/1 -> Minus11/2
  Cos8/1 -> Product16/2
  Constant59/1 -> Product6/2
  VWRL/1 -> V_WRL/1
  Product5/1 -> VWFR/2
  Constant60/1 -> Product17/1
  Cos7/1 -> Product4/1
  Product14/1 -> Minus10/1
  Cos5/1 -> Product1/1
  VWRR/1 -> V_WRR/1
  wsz/1 -> Gain45/1
  Constant61/1 -> Product8/2
  Cos4/1 -> Product14/2
  Cos10/1 -> Product17/2
  Cos6/1 -> Product15/2
  Minus13/1 -> Product9/2
  Constant58/1 -> Product16/1
  Constant54/1 -> Product14/1
  Product3/1 -> VWFL/2
  Minus11/1 -> Product5/2
  Product8/1 -> Minus13/2
  Product17/1 -> Minus13/1
  VWFL/1 -> V_WFL/1
  Product9/1 -> VWRR/2
  Constant55/1 -> Product1/2
  Cos11/1 -> Product8/1
  Product15/1 -> Minus11/1
  Minus10/1 -> Product3/2
  Product7/1 -> VWRL/2
  beta/1 -> Cos8/1, Cos9/1, Cos11/1, Cos10/1, Cos7/1, Cos6/1, Cos4/1, Cos5/1
  Gain45/1 -> Product9/1, Product7/1, Product5/1, Product3/1
  vcog/1 -> VWRR/1, VWRL/1, VWFR/1, VWFL/1

== system vehiclemodel_simple_empty_2020a/Subsystem2/Subsystem4 ==
  Fwz : Inport
  B : Inport  Port=2
  C : Inport  Port=3
  D : Inport  Port=4
  E : Inport  Port=5
  kappa : Inport  Port=6
  alpha : Inport  Port=7
  Fx : Outport
  Fy : Outport  Port=2

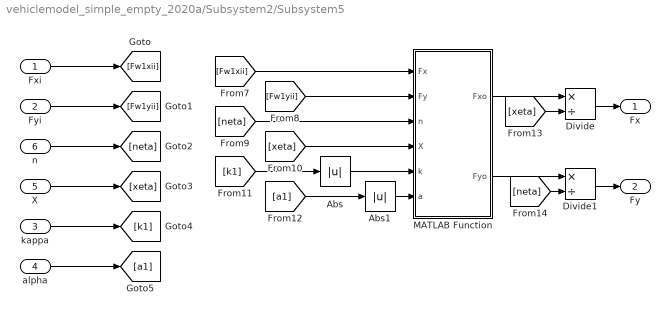
== system vehiclemodel_simple_empty_2020a/Subsystem2/Subsystem5 ==
  Fxi : Inport
  Fyi : Inport  Port=2
  kappa : Inport  Port=3
  alpha : Inport  Port=4
  X : Inport  Port=5
  n : Inport  Port=6
  Abs : Abs  SaturateOnIntegerOverflow=off
  Abs1 : Abs  SaturateOnIntegerOverflow=off
  Divide : Product  Inputs=*/
  Divide1 : Product  Inputs=*/
  MATLAB Function : MATLAB Function  TreatAsAtomicUnit=on
  Fx : Outport
  Fy : Outport  Port=2
  wires:
  Divide1/1 -> Fy/1
  [neta] -> Divide1/2
  MATLAB Function/2(Fyo) -> Divide1/1
  Abs/1 -> MATLAB Function/5(k)
  [xeta] -> Divide/2
  [a1] -> Abs1/1
  [xeta] -> MATLAB Function/4(X)
  Abs1/1 -> MATLAB Function/6(a)
  MATLAB Function/1(Fxo) -> Divide/1
  [Fw1yii] -> MATLAB Function/2(Fy)
  [neta] -> MATLAB Function/3(n)
  [k1] -> Abs/1
  [Fw1xii] -> MATLAB Function/1(Fx)
  Divide/1 -> Fx/1
  kappa/1 -> [k1]
  alpha/1 -> [a1]
  X/1 -> [xeta]
  n/1 -> [neta]
  Fyi/1 -> [Fw1yii]
  Fxi/1 -> [Fw1xii]

== system vehiclemodel_simple_empty_2020a/Subsystem2/Subsystem6 ==
  Fwz : Inport
  B : Inport  Port=2
  C : Inport  Port=3
  D : Inport  Port=4
  E : Inport  Port=5
  kappa : Inport  Port=6
  alpha : Inport  Port=7
  Fx : Outport
  Fy : Outport  Port=2

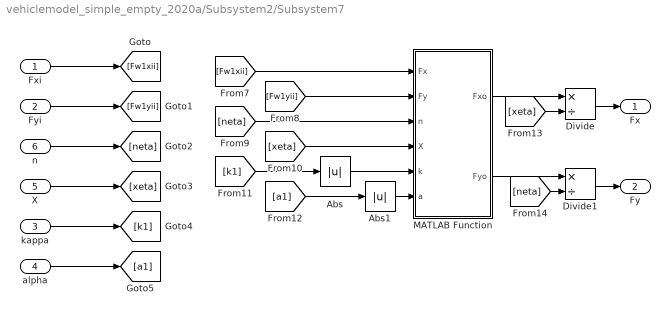
== system vehiclemodel_simple_empty_2020a/Subsystem2/Subsystem7 ==
  Fxi : Inport
  Fyi : Inport  Port=2
  kappa : Inport  Port=3
  alpha : Inport  Port=4
  X : Inport  Port=5
  n : Inport  Port=6
  Abs : Abs  SaturateOnIntegerOverflow=off
  Abs1 : Abs  SaturateOnIntegerOverflow=off
  Divide : Product  Inputs=*/
  Divide1 : Product  Inputs=*/
  MATLAB Function : MATLAB Function  TreatAsAtomicUnit=on
  Fx : Outport
  Fy : Outport  Port=2
  wires:
  Divide1/1 -> Fy/1
  [neta] -> Divide1/2
  MATLAB Function/2(Fyo) -> Divide1/1
  Abs/1 -> MATLAB Function/5(k)
  [xeta] -> Divide/2
  [a1] -> Abs1/1
  [xeta] -> MATLAB Function/4(X)
  Abs1/1 -> MATLAB Function/6(a)
  MATLAB Function/1(Fxo) -> Divide/1
  [Fw1yii] -> MATLAB Function/2(Fy)
  [neta] -> MATLAB Function/3(n)
  [k1] -> Abs/1
  [Fw1xii] -> MATLAB Function/1(Fx)
  Divide/1 -> Fx/1
  kappa/1 -> [k1]
  alpha/1 -> [a1]
  X/1 -> [xeta]
  n/1 -> [neta]
  Fyi/1 -> [Fw1yii]
  Fxi/1 -> [Fw1xii]

== system vehiclemodel_simple_empty_2020a/Subsystem2/Subsystem8 ==
  Fwz : Inport
  B : Inport  Port=2
  C : Inport  Port=3
  D : Inport  Port=4
  E : Inport  Port=5
  kappa : Inport  Port=6
  alpha : Inport  Port=7
  Fx : Outport
  Fy : Outport  Port=2

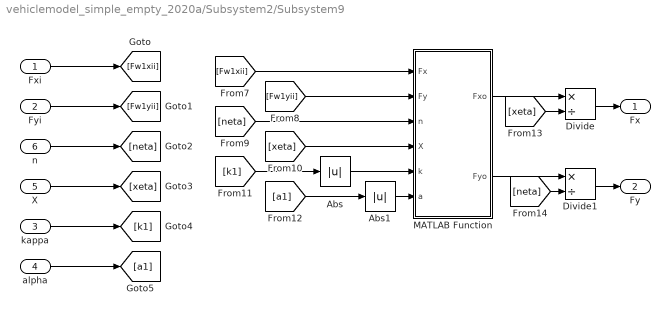
== system vehiclemodel_simple_empty_2020a/Subsystem2/Subsystem9 ==
  Fxi : Inport
  Fyi : Inport  Port=2
  kappa : Inport  Port=3
  alpha : Inport  Port=4
  X : Inport  Port=5
  n : Inport  Port=6
  Abs : Abs  SaturateOnIntegerOverflow=off
  Abs1 : Abs  SaturateOnIntegerOverflow=off
  Divide : Product  Inputs=*/
  Divide1 : Product  Inputs=*/
  MATLAB Function : MATLAB Function  TreatAsAtomicUnit=on
  Fx : Outport
  Fy : Outport  Port=2
  wires:
  Fxi/1 -> [Fw1xii]
  Fyi/1 -> [Fw1yii]
  n/1 -> [neta]
  X/1 -> [xeta]
  alpha/1 -> [a1]
  kappa/1 -> [k1]
  Divide/1 -> Fx/1
  [Fw1xii] -> MATLAB Function/1(Fx)
  [k1] -> Abs/1
  [neta] -> MATLAB Function/3(n)
  [Fw1yii] -> MATLAB Function/2(Fy)
  MATLAB Function/1(Fxo) -> Divide/1
  Abs1/1 -> MATLAB Function/6(a)
  [xeta] -> MATLAB Function/4(X)
  [a1] -> Abs1/1
  [xeta] -> Divide/2
  Abs/1 -> MATLAB Function/5(k)
  MATLAB Function/2(Fyo) -> Divide1/1
  [neta] -> Divide1/2
  Divide1/1 -> Fy/1

== system vehiclemodel_simple_empty_2020a/Subsystem/Acceleration Based Algorithm/Subsystem1 ==
  A : Inport
  Command : Outport

== system vehiclemodel_simple_empty_2020a/Subsystem/Acceleration Based Algorithm/Subsystem2 ==
  A : Inport
  Command : Outport

== system vehiclemodel_simple_empty_2020a/Subsystem/Acceleration Based Algorithm/Subsystem3 ==
  A : Inport
  Command : Outport

== system vehiclemodel_simple_empty_2020a/Subsystem/Acceleration Based Algorithm/Subsystem4 ==
  A : Inport
  Command : Outport

== system vehiclemodel_simple_empty_2020a/Subsystem/Slip Based Algorithm/Subsystem1 ==
  A : Inport
  Command : Outport

== system vehiclemodel_simple_empty_2020a/Subsystem/Slip Based Algorithm/Subsystem2 ==
  A : Inport
  Command : Outport

== system vehiclemodel_simple_empty_2020a/Subsystem/Slip Based Algorithm/Subsystem3 ==
  A : Inport
  Command : Outport

== system vehiclemodel_simple_empty_2020a/Subsystem/Slip Based Algorithm/Subsystem4 ==
  A : Inport
  Command : Outport

== matlab function vehiclemodel_simple_empty_2020a/Subsystem2/Subsystem9/MATLAB Function ==
  data: Fx input; Fxo output; Fy input; n input; X input; k input; a input; Fyo output
function [Fxo,Fyo] = fcn(Fx,Fy,n,X,k,a)

Fxo = Fx*(X/((X*(a^2))+1));

Fyo = Fy*(n/((n*(k^2))+1));

== matlab function vehiclemodel_simple_empty_2020a/MATLAB Function ==
  data: H input; Lw output; L input; S input; sig input; Rw output
function [Lw,Rw] = fcn(H,L,S,sig)

Lw = H;
Rw = H;

if sig == 1
    Lw = H;
    Rw = H;
end

if sig == 2
    Lw = L;
    Rw = L;
end

if sig == 3
    Lw = L;
    Rw = H;
end

if sig == 4
    if S < 40
        Lw = H;
        Rw = H;
    else
        Lw = L;
        Rw = L;
    end
end

if sig == 5
    Lw = H;
    Rw = H;
    if S < 90
        Lw = H;
        Rw = L;
    end
    if S < 80
        Lw = L;
        Rw = H;
    end
    if S < 70
        Lw = H;
        Rw = L;
    end
    if S < 60
        Lw = L;
        Rw = H;
    end
    if S < 50
        Lw = H;
        Rw = L;
    end
    if S < 40
        Lw = L;
        Rw = H;
    end
    if S < 30
        Lw = H;
        Rw = L;
    end
end

== matlab function vehiclemodel_simple_empty_2020a/Subsystem2/Subsystem7/MATLAB Function ==
  data: Fx input; Fxo output; Fy input; n input; X input; k input; a input; Fyo output
function [Fxo,Fyo] = fcn(Fx,Fy,n,X,k,a)

Fxo = Fx*(X/((X*(a^2))+1));

Fyo = Fy*(n/((n*(k^2))+1));

== matlab function vehiclemodel_simple_empty_2020a/Subsystem2/Brake Torque Calculation ==
  data: BP input; Tb1 output; Po input; Ab input; BF input; nm input; p input; fa input; ff input; r input; Tb2 output; Tb3 output; Tb4 output
function [Tb1,Tb2,Tb3,Tb4] = fcn(BP,Po,Ab,BF,nm,p,fa,ff,r)

    Tb1 = ((BP(1))-(Po+101325))*Ab*BF*nm*p*fa*ff*r;

    Tb2 = ((BP(2))-(Po+101325))*Ab*BF*nm*p*fa*ff*r;

    Tb3 = ((BP(3))-(Po+101325))*Ab*BF*nm*p*fa*ff*r;

    Tb4 = ((BP(4))-(Po+101325))*Ab*BF*nm*p*fa*ff*r;

== matlab function vehiclemodel_simple_empty_2020a/Subsystem/Slip Based Algorithm/MATLAB Function2 ==
  data: BP1 input; y1 output; BP2 input; y2 output; y3 output; y4 output; BP3 input; BP4 input; V input; ABS input
function [y1,y2,y3,y4] = fcn(BP1,BP2,BP3,BP4,V,ABS)

y1 = BP1;
y2 = BP2;
y3 = BP3;
y4 = BP4;

if V < 2
    y1 = 1;
    y2 = 1;
    y3 = 1;
    y4 = 1;
end

if ABS == 0
    y1 = 1;
    y2 = 1;
    y3 = 1;
    y4 = 1;
end

== matlab function vehiclemodel_simple_empty_2020a/Subsystem/Acceleration Based Algorithm/MATLAB Function2 ==
  data: BP1 input; y1 output; BP2 input; y2 output; y3 output; y4 output; BP3 input; BP4 input; V input; ABS input
function [y1,y2,y3,y4] = fcn(BP1,BP2,BP3,BP4,V,ABS)

y1 = BP1;
y2 = BP2;
y3 = BP3;
y4 = BP4;

if V < 2
    y1 = 1;
    y2 = 1;
    y3 = 1;
    y4 = 1;
end

if ABS == 0
    y1 = 1;
    y2 = 1;
    y3 = 1;
    y4 = 1;
end

== matlab function vehiclemodel_simple_empty_2020a/Subsystem/ABS Safety ==
  data: Fp input; y output
function y = fcn(Fp)

if Fp > 0
    y = 1;
else
    y = 2;
end

== matlab function vehiclemodel_simple_empty_2020a/Subsystem2/Subsystem2/MATLAB Function ==
  data: Fx input; Fxo output; Fy input; n input; X input; k input; a input; Fyo output
function [Fxo,Fyo] = fcn(Fx,Fy,n,X,k,a)

Fxo = Fx*(X/((X*(a^2))+1));

Fyo = Fy*(n/((n*(k^2))+1));

== matlab function vehiclemodel_simple_empty_2020a/Subsystem2/Subsystem5/MATLAB Function ==
  data: Fx input; Fxo output; Fy input; n input; X input; k input; a input; Fyo output
function [Fxo,Fyo] = fcn(Fx,Fy,n,X,k,a)

Fxo = Fx*(X/((X*(a^2))+1));

Fyo = Fy*(n/((n*(k^2))+1));
